simulink model "ACDCMG_woPV"  (R2020b)
settings: Solver=FixedStepAuto  StartTime=0.0  StopTime=0.2  FixedStep=Ts  MaxStep=1e-2  RelTol=1e-3
InitFcn:
  | Set_parameters_R2018
undefined symbols (not defined in the file): D1, D_invs, Delta, dis11, dis14, dis2, dis3, dis4, dis5, dis6, dis8, DiscIntNeverNeededParam, ee_sli_rtmsupport, fn, Fnom, gcbh, H_invs, Ion, Lithium, max_min, P_Load_3, P_nom_inv, Pnom_T1, Pnom_T2, Pnom_T3, Ql_Load_3, R_Load_9, R_Load_DC, Rl, Rls, S, sigbuilder_block, Ts, Ts_Control, Ts_Power, V1_LL_T3, VnInv, Vnom_DC, Vnom_Diesel, Vnom_prim, Vnom_sec, Vnom_ter_AC_DC, Xl, Xls
libraries: powerlib x238, powerlib_meascontrol x103, powerlib_extras x55, simulink x21, pid_lib x4, eeGeneralControl x2, re_lib x1, electricdrivelib x1, eeSinusoidalMeasurementV2 x1, eePowerMeasurement x1
(part 7 of 9)

== system ACDCMG_woPV/Inverter 300 (DC) // 150 V (AC) P_nom 3kW4/Control of Inverter/Positive-Sequence Active & Reactive Power1 ==
  note: Discrete 3-phase Positive-Sequence Active & Reactive Power
  note: Pierre Giroux, Gilbert Sybille
      | Power System Simulation Laboratory
      | IREQ, Hydro-Quebc
  Vabc : Inport  PortDimensions=3
  Iabc : Inport  Port=2  PortDimensions=3
  Deg->Rad : Gain  Gain=pi/180  SaturateOnIntegerOverflow=on  OutDataTypeStr=Inherit: Same as input  ParamDataTypeStr=Inherit: Same as input
  Discrete 3-phase Positive-Sequence Fundamental Value (I) : powerlib_extras/Discrete Measurements/Discrete 3-phase Positive-Sequence Fundamental Value  Freq=Freq  Par_Init=Par_Iinit  Ts=Ts
      settings: SourceProductBaseCode=PS
  Discrete 3-phase Positive-Sequence Fundamental Value (V) : powerlib_extras/Discrete Measurements/Discrete 3-phase Positive-Sequence Fundamental Value  Freq=Freq  Par_Init=Par_Vinit  Ts=Ts
      settings: SourceProductBaseCode=PS
  Gain1 : Gain  Gain=3/2  SaturateOnIntegerOverflow=on  OutDataTypeStr=Inherit: Same as input  ParamDataTypeStr=Inherit: Same as input
  Mag->RMS : Gain  Gain=1/sqrt(2)
  Mux1 : Mux  Inputs=2
  Mux2 : Mux  Inputs=2
  Mux3 : Mux  Inputs=2
  Product : Product  InputSameDT=on  SaturateOnIntegerOverflow=on  OutDataTypeStr=Inherit: Same as first input
  Product1 : Product  InputSameDT=on  SaturateOnIntegerOverflow=on  OutDataTypeStr=Inherit: Same as first input
  Product2 : Product  InputSameDT=on  SaturateOnIntegerOverflow=on  OutDataTypeStr=Inherit: Same as first input
  Sum : Sum  Inputs=+-  InputSameDT=on  SaturateOnIntegerOverflow=on  OutDataTypeStr=Inherit: Same as first input
  Trigonometric Function : Trigonometry
  Trigonometric Function1 : Trigonometry  Operator=cos
  W->kW Var->kvar : Gain  Gain=1/1000
  RMS_V_I : Outport
  P_Q(kW) : Outport  Port=2
  Phase_V_I : Outport  Port=3
  PF : Outport  Port=4
  wires:
  Vabc/1 -> Discrete 3-phase Positive-Sequence Fundamental Value (V)/1
  Iabc/1 -> Discrete 3-phase Positive-Sequence Fundamental Value (I)/1
  Discrete 3-phase Positive-Sequence Fundamental Value (V)/2 -> Sum/1, Mux1/1
  Discrete 3-phase Positive-Sequence Fundamental Value (I)/2 -> Sum/2, Mux1/2
  Sum/1 -> Deg->Rad/1
  Deg->Rad/1 -> Trigonometric Function1/1, Trigonometric Function/1
  Trigonometric Function1/1 -> PF/1, Product/2
  Trigonometric Function/1 -> Product1/1
  Mux2/1 -> Gain1/1
  Product/1 -> Mux2/1
  Product1/1 -> Mux2/2
  Product2/1 -> Product/1, Product1/2
  Discrete 3-phase Positive-Sequence Fundamental Value (V)/1 -> Mux3/1, Product2/1
  Discrete 3-phase Positive-Sequence Fundamental Value (I)/1 -> Mux3/2, Product2/2
  Mux1/1 -> Phase_V_I/1
  Mux3/1 -> Mag->RMS/1
  Mag->RMS/1 -> RMS_V_I/1
  Gain1/1 -> W->kW Var->kvar/1
  W->kW Var->kvar/1 -> P_Q(kW)/1

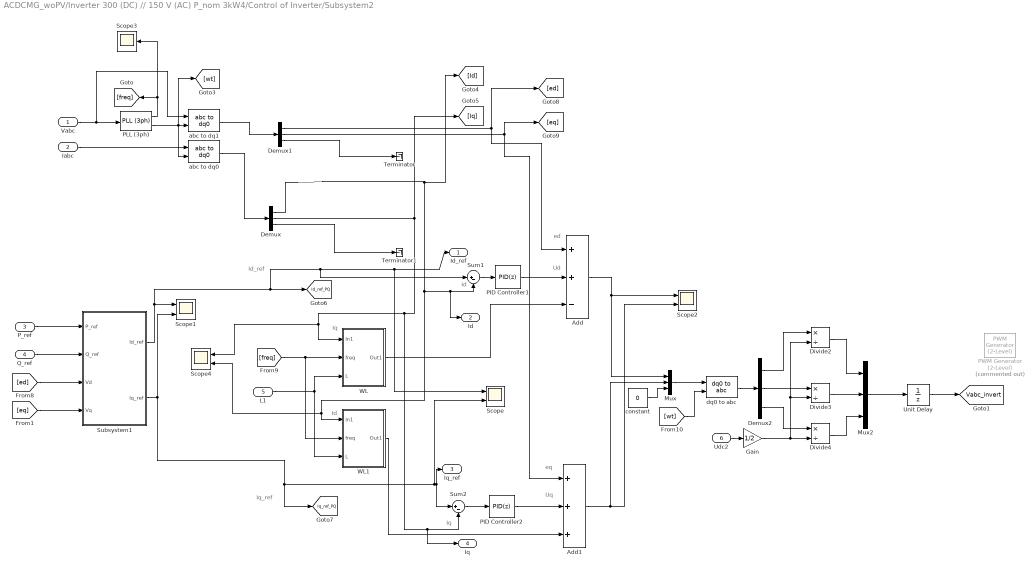
== system ACDCMG_woPV/Inverter 300 (DC) // 150 V (AC) P_nom 3kW4/Control of Inverter/Subsystem2 ==
  note: Iq_ref
  note: Id
  note: Id_ref
  note: Ud
  note: Uq
  note: eq
  note: ed
  note: Iq
  note: Id
  note: Iq
  Vabc : Inport
  Iabc : Inport  Port=2
  P_ref : Inport  Port=3
  Q_ref : Inport  Port=4
  L1 : Inport  Port=5
  Udc2 : Inport  Port=6
  Add : Sum  Inputs=++-
  Add1 : Sum  Inputs=+++
  Demux : Demux  Outputs=3
  Demux1 : Demux  Outputs=3
  Demux2 : Demux  Outputs=3
  Divide2 : Product  Inputs=*/
  Divide3 : Product  Inputs=*/
  Divide4 : Product  Inputs=*/
  Gain : Gain  Gain=1/2
  Mux : Mux  Inputs=3
  Mux2 : Mux  Inputs=3
  PID Controller1 : pid_lib/PID Controller  Controller=PID  Form=Parallel  TimeDomain=Discrete-time  UseExternalTs=off  SampleTime=Ts_Control  IntegratorMethod=Forward Euler  FilterMethod=Forward Euler  ControllerParametersSource=internal  P=Kp  I=Ki  D=Kd  N=100  UseFilter=on  TunerSelectOption=Transfer Function Based (PID Tuner App)  InitialConditionSource=internal  InitialConditionForIntegrator=0  InitialConditionForFilter=0  DifferentiatorICPrevScaledInput=0  ExternalReset=none  TrackingMode=off  Kt=1  LimitOutput=off  SatLimitsSource=internal  UpperSaturationLimit=inf  LowerSaturationLimit=-inf  LinearizeAsGain=on  AntiWindupMode=none  Kb=1  POutMin=[]  POutMax=[]  IOutMin=[]  IOutMax=[]  DOutMin=[]  DOutMax=[]  NOutMin=[]  NOutMax=[]  SumOutMin=[]  SumOutMax=[]  SaturationOutMin=[]  SaturationOutMax=[]  PParamMin=[]  PParamMax=[]  IParamMin=[]  IParamMax=[]  DParamMin=[]  DParamMax=[]  NParamMin=[]  NParamMax=[]  KbParamMin=[]  KbParamMax=[]  KtParamMin=[]  KtParamMax=[]  KbOutMin=[]  KbOutMax=[]  KtOutMin=[]  KtOutMax=[]  IntegratorOutMin=[]  IntegratorOutMax=[]  FilterOutMin=[]  FilterOutMax=[]  SumI1OutMin=[]  SumI1OutMax=[]  SumI2OutMin=[]  SumI2OutMax=[]  SumI3OutMin=[]  SumI3OutMax=[]  SumI4OutMin=[]  SumI4OutMax=[]  SumDOutMin=[]  SumDOutMax=[]  DifferentiatorOutMin=[]  DifferentiatorOutMax=[]  FilterDiffOutCoefMin=[]  FilterDiffOutCoefMax=[]  ReciprocalOutMin=[]  ReciprocalOutMax=[]  SumDenOutMin=[]  SumDenOutMax=[]  SumNumOutMin=[]  SumNumOutMax=[]  DivideOutMin=[]  DivideOutMax=[]  UdiffTsProdOutMin=[]  UdiffTsProdOutMax=[]  NTsProdOutMin=[]  NTsProdOutMax=[]  UintegralTsProdOutMin=[]  UintegralTsProdOutMax=[]  UngainTsProdOutMin=[]  UngainTsProdOutMax=[]  IntegratorContinuousStateAttributes=''  IntegratorStateMustResolveToSignalObject=off  IntegratorRTWStateStorageClass=Auto  FilterContinuousStateAttributes=''  FilterStateMustResolveToSignalObject=off  FilterRTWStateStorageClass=Auto  ParallelPVariant=InternalParameters  IdealPVariant=Disabled  IVariant=InternalParameters  DVariant=InternalParameters  IntegratorVariant=Discrete  SatVariant=Disabled  AWVariant=Passthrough  PCopyVariant=Disabled  TRVariant=Disabled  FdbkBlocksVariant=Forward  IdealPFdbkVariant=Disabled  SatFdbkVariant=Disabled  DerivativeFilterVariant=ForwardEulerFilter  NVariant=InternalParameters  NCopyVariant=Disabled  FilterICVariant=InternalICsFilter  IntegratorICVariant=InternalICs  ExternalResetVariant=Disabled  TRSumVariant=Passthrough  SumFdbkVariant=Disabled  SumVariant=Sum_PID  TsampFilterVariant=InternalTs  TsampNgainVariant=Passthrough  TsampIntegralVariant=Passthrough  ExternalSaturationOutDataTypeStr=Inherit: Same as second input
  PID Controller2 : pid_lib/PID Controller  Controller=PID  Form=Parallel  TimeDomain=Discrete-time  UseExternalTs=off  SampleTime=Ts_Control  IntegratorMethod=Forward Euler  FilterMethod=Forward Euler  ControllerParametersSource=internal  P=Kp  I=Ki  D=Kd  N=100  UseFilter=on  TunerSelectOption=Transfer Function Based (PID Tuner App)  InitialConditionSource=internal  InitialConditionForIntegrator=0  InitialConditionForFilter=0  DifferentiatorICPrevScaledInput=0  ExternalReset=none  TrackingMode=off  Kt=1  LimitOutput=off  SatLimitsSource=internal  UpperSaturationLimit=inf  LowerSaturationLimit=-inf  LinearizeAsGain=on  AntiWindupMode=none  Kb=1  POutMin=[]  POutMax=[]  IOutMin=[]  IOutMax=[]  DOutMin=[]  DOutMax=[]  NOutMin=[]  NOutMax=[]  SumOutMin=[]  SumOutMax=[]  SaturationOutMin=[]  SaturationOutMax=[]  PParamMin=[]  PParamMax=[]  IParamMin=[]  IParamMax=[]  DParamMin=[]  DParamMax=[]  NParamMin=[]  NParamMax=[]  KbParamMin=[]  KbParamMax=[]  KtParamMin=[]  KtParamMax=[]  KbOutMin=[]  KbOutMax=[]  KtOutMin=[]  KtOutMax=[]  IntegratorOutMin=[]  IntegratorOutMax=[]  FilterOutMin=[]  FilterOutMax=[]  SumI1OutMin=[]  SumI1OutMax=[]  SumI2OutMin=[]  SumI2OutMax=[]  SumI3OutMin=[]  SumI3OutMax=[]  SumI4OutMin=[]  SumI4OutMax=[]  SumDOutMin=[]  SumDOutMax=[]  DifferentiatorOutMin=[]  DifferentiatorOutMax=[]  FilterDiffOutCoefMin=[]  FilterDiffOutCoefMax=[]  ReciprocalOutMin=[]  ReciprocalOutMax=[]  SumDenOutMin=[]  SumDenOutMax=[]  SumNumOutMin=[]  SumNumOutMax=[]  DivideOutMin=[]  DivideOutMax=[]  UdiffTsProdOutMin=[]  UdiffTsProdOutMax=[]  NTsProdOutMin=[]  NTsProdOutMax=[]  UintegralTsProdOutMin=[]  UintegralTsProdOutMax=[]  UngainTsProdOutMin=[]  UngainTsProdOutMax=[]  IntegratorContinuousStateAttributes=''  IntegratorStateMustResolveToSignalObject=off  IntegratorRTWStateStorageClass=Auto  FilterContinuousStateAttributes=''  FilterStateMustResolveToSignalObject=off  FilterRTWStateStorageClass=Auto  ParallelPVariant=InternalParameters  IdealPVariant=Disabled  IVariant=InternalParameters  DVariant=InternalParameters  IntegratorVariant=Discrete  SatVariant=Disabled  AWVariant=Passthrough  PCopyVariant=Disabled  TRVariant=Disabled  FdbkBlocksVariant=Forward  IdealPFdbkVariant=Disabled  SatFdbkVariant=Disabled  DerivativeFilterVariant=ForwardEulerFilter  NVariant=InternalParameters  NCopyVariant=Disabled  FilterICVariant=InternalICsFilter  IntegratorICVariant=InternalICs  ExternalResetVariant=Disabled  TRSumVariant=Passthrough  SumFdbkVariant=Disabled  SumVariant=Sum_PID  TsampFilterVariant=InternalTs  TsampNgainVariant=Passthrough  TsampIntegralVariant=Passthrough  ExternalSaturationOutDataTypeStr=Inherit: Same as second input
  PLL (3ph) : powerlib_meascontrol/PLL/PLL (3ph)  Fmin=59.5  Par_Init=[0, 60]  ParK=[180, 3200, 1]  TcD=1e-4  MaxRateChangeFreq=12  FilterCutOffFreq=25  Ts=Ts_Control  AGC=on
  PWM Generator (2-Level) : powerlib_meascontrol/Pulse & Signal Generators/PWM Generator (2-Level)  Commented=on  ModulatorType=Three-phase bridge (6 pulses)  ModulatorMode=Unsynchronized  Fc=15000  Pc=90  nF=27  MinMax="[ -1  1 ]"  SamplingTechnique=Natural  ModulatingSignals=off  m=0.8  Freq=60  Phase=0  Ts=Ts_Power  ShowCarrierOutport=off
  Scope{,1..2,4} (4 alike) : Scope  NumInputPorts=2
  Scope3 : Scope
  Subsystem1 : Subsystem
  Sum1 : Sum  Inputs=|+-
  Sum2 : Sum  Inputs=|+-
  Terminator : Terminator
  Terminator1 : Terminator
  Unit Delay : UnitDelay  SampleTime=-1  HasFrameUpgradeWarning=on
  WL : Subsystem
  WL1 : Subsystem
  abc to dq0 : powerlib_meascontrol/Transformations/abc to dq0  Alignment=90 degrees behind phase A axis
  abc to dq1 : powerlib_meascontrol/Transformations/abc to dq0  Alignment=90 degrees behind phase A axis
  constant : Constant  Value=0
  dq0 to abc : powerlib_meascontrol/Transformations/dq0 to abc  Alignment=90 degrees behind phase A axis
  Id_ref : Outport
  Id : Outport  Port=2
  Iq_ref : Outport  Port=3
  Iq : Outport  Port=4
  tag scope: Id_ref_PQ=global, Iq_ref_PQ=global, Vabc_invert=global
  wires:
  abc to dq1/1 -> Demux1/1
  Sum1/1 -> PID Controller1/1
  Iabc/1 -> abc to dq0/1
  Vabc/1 -> abc to dq1/1, PLL (3ph)/1
  PLL (3ph)/2 -> [wt], abc to dq1/2, abc to dq0/2
  Demux1/1 -> Add/1, [ed]
  L1/1 -> WL/3(L), WL1/3(L)
  WL/1(Out1) -> Add/3
  [freq] -> WL1/2(freq), WL/2(freq)
  PLL (3ph)/1 -> Scope3/1, [freq]
  Demux2/1 -> Divide2/1
  Add/1 -> Mux/1, Scope2/1
  PID Controller2/1 -> Add1/2
  Sum2/1 -> PID Controller2/1
  Demux2/2 -> Divide3/1
  WL1/1(Out1) -> Add1/3
  Demux1/2 -> Add1/1, [eq]
  Add1/1 -> Mux/2, Scope2/2
  Gain/1 -> Divide3/2, Divide2/2, Divide4/2
  Divide4/1 -> Mux2/3
  Divide2/1 -> Mux2/1
  Mux/1 -> dq0 to abc/1
  Demux2/3 -> Divide4/1
  Divide3/1 -> Mux2/2
  dq0 to abc/1 -> Demux2/1
  PID Controller1/1 -> Add/2
  [wt] -> dq0 to abc/2
  Udc2/1 -> Gain/1
  Demux1/3 -> Terminator/1
  Demux/3 -> Terminator1/1
  constant/1 -> Mux/3
  P_ref/1 -> Subsystem1/1(P_ref)
  Q_ref/1 -> Subsystem1/2(Q_ref)
  [ed] -> Subsystem1/3(Vd)
  [eq] -> Subsystem1/4(Vq)
  Subsystem1/2(Iq_ref) -> Scope1/2, [Iq_ref_PQ], Scope/2, Iq_ref/1, Sum2/1
  Subsystem1/1(Id_ref) -> Sum1/1, Scope/1, Id_ref/1, [Id_ref_PQ], Scope1/1
  Demux/1 -> Scope4/2, WL1/1(In1), Id/1, Sum1/2, [Id]
  Demux/2 -> [Iq], Scope4/1, WL/1(In1), Iq/1, Sum2/2
  abc to dq0/1 -> Demux/1
  Mux2/1 -> Unit Delay/1
  Unit Delay/1 -> [Vabc_invert]

== system ACDCMG_woPV/Inverter 300 (DC) // 150 V (AC) P_nom 3kW4/Control of Inverter/V//F ==
  e : Inport
  io : Inport  Port=2
  i : Inport  Port=3
  Udc : Inport  Port=4
  Constant : Constant  Value=150*sqrt(2)
  Constant1 : Constant  Value=0
  Constant2 : Constant  Commented=on
  Constant3 : Constant  Commented=on
  Constant4 : Constant
  From : From  Commented=on  GotoTag=P_mea_inv  TagVisibility=global
  Gain : Gain  Commented=on  Gain=1/P_nom_inv
  Gain1 : Gain  Gain=Fnom
  Gain2 : Gain  Commented=on  Gain=-1
  Scope : Scope  NumInputPorts=2
  Subsystem : Subsystem
  Sum : Sum  Commented=on  Inputs=|+-
  Sum1 : Sum  Commented=on  Inputs=|++
  Transfer Fcn : TransferFcn  Commented=on  Denominator=[2*H_invs D_invs]
  UIcontrol : Subsystem
  wires:
  Constant/1 -> UIcontrol/1(ed_ref)
  Constant1/1 -> UIcontrol/3(eq_ref)
  Udc/1 -> UIcontrol/9(Udc)
  e/1 -> Subsystem/1(e)
  i/1 -> Subsystem/3(i)
  Subsystem/1(ed) -> UIcontrol/2(ed)
  Subsystem/2(eq) -> UIcontrol/4(eq)
  Subsystem/3(iod) -> UIcontrol/5(iod)
  Subsystem/4(ioq) -> UIcontrol/6(ioq)
  Subsystem/8("wt ") -> UIcontrol/8("wt ")
  Subsystem/7(w) -> UIcontrol/7(w)
  Subsystem/5(id) -> UIcontrol/11(id)
  Subsystem/6(iq) -> UIcontrol/10(iq)
  io/1 -> Subsystem/2(io)
  From/1 -> Gain/1
  Gain1/1 -> Scope/1, Subsystem/4(fcmd)
  Gain/1 -> Scope/2, Sum/1
  Constant2/1 -> Sum/2
  Sum/1 -> Gain2/1
  Gain2/1 -> Transfer Fcn/1
  Transfer Fcn/1 -> Sum1/1
  Constant3/1 -> Sum1/2
  Constant4/1 -> Gain1/1

== system ACDCMG_woPV/Grid Bi-directional Converter 1.1 300 (DC) // 150 V (AC) P_nom 3kW/Control of Inverter/MI Controller/OP max // min ==
  note: DC to AC
  note: AC to DC
  Constant2 : Constant  Value=max_min
  OP_max1 : Constant  Value=1.2
  OP_min1 : Constant
  Switch2 : Switch  Criteria=u2 > Threshold
  ctrl : Outport  VectorParamsAs1DForOutWhenUnconnected=off
  wires:
  OP_max1/1 -> Switch2/1
  OP_min1/1 -> Switch2/3
  Constant2/1 -> Switch2/2
  Switch2/1 -> ctrl/1

== system ACDCMG_woPV/Grid Bi-directional Converter 1.1 300 (DC) // 150 V (AC) P_nom 3kW/Control of Inverter/MI Controller/Subsystem ==
  sin_cos : Inport  PortDimensions=2
  Demux : Demux  Outputs=2
      settings: DisplayOption=none
  Fcn2 : Fcn  Expr=1*u[1]
  Fcn4 : Fcn  Expr=1*u[3]
  Fcn5 : Fcn  Expr=1*u[5]
  K1 : Constant  Value=0.5
  K2 : Constant  Value=sqrt(3)/2
  Mux2 : Mux  Inputs=6
  Product{,1..3} (4 alike) : Product  InputSameDT=on  SaturateOnIntegerOverflow=on  OutDataTypeStr=Inherit: Same as first input
  Sum : Sum  Inputs=--  InputSameDT=on  SaturateOnIntegerOverflow=on  OutDataTypeStr=Inherit: Same as first input
  Sum1 : Sum  Inputs=-+  InputSameDT=on  SaturateOnIntegerOverflow=on  OutDataTypeStr=Inherit: Same as first input
  Sum2 : Sum  Inputs=--  InputSameDT=on  SaturateOnIntegerOverflow=on  OutDataTypeStr=Inherit: Same as first input
  Sum3 : Sum  Inputs=--  InputSameDT=on  SaturateOnIntegerOverflow=on  OutDataTypeStr=Inherit: Same as first input
  Va : Outport  VectorParamsAs1DForOutWhenUnconnected=off
  Vb : Outport  Port=2  VectorParamsAs1DForOutWhenUnconnected=off
  Vc : Outport  Port=3  VectorParamsAs1DForOutWhenUnconnected=off
  wires:
  sin_cos/1 -> Demux/1
  Demux/1 -> Product/1, Product2/1, Sum2/2, Mux2/1  "sin(wt)"
  Product/1 -> Sum/1
  Product1/1 -> Sum/2
  Product3/1 -> Sum1/1
  Product2/1 -> Sum1/2
  Sum3/1 -> Mux2/6  "cos(wt+2pi/3)"
  Sum2/1 -> Mux2/5  "sin(wt+2pi/3)"
  K1/1 -> Product/2, Product3/2
  K2/1 -> Product1/2, Product2/2
  Sum/1 -> Mux2/3, Sum2/1  "sin(wt-2pi/3)"
  Sum1/1 -> Mux2/4, Sum3/1  "cos(wt-2pi/3)"
  Demux/2 -> Sum3/2, Product3/1, Product1/1, Mux2/2  "cos(wt)"
  Mux2/1 -> Fcn2/1, Fcn4/1, Fcn5/1
  Fcn2/1 -> Va/1
  Fcn4/1 -> Vb/1
  Fcn5/1 -> Vc/1

== system ACDCMG_woPV/Grid Bi-directional Converter 1.1 300 (DC) // 150 V (AC) P_nom 3kW/Control of Inverter/MI Controller/Subsystem1 ==
  note: AC to DC
  note: DC to AC
  Constant1 : Constant  Value=max_min
  Constant2 : Constant  Value=2*pi
  Deg->Rad : Gain  Gain=pi/180  SaturateOnIntegerOverflow=on  OutDataTypeStr=Inherit: Same as input  ParamDataTypeStr=Inherit: Same as input
  Freq1 : Constant  Value=Fnom
  Freq2 : Constant  Value=2*pi
  Math Function : Math  Operator=mod  SignedPower=on  SaturateOnIntegerOverflow=on
  Mux5 : Mux  Inputs=2
  OP_max1 : Constant  Value=0
  OP_min1 : Constant  Value=228
  Product7 : Product  Inputs=***  InputSameDT=on  SaturateOnIntegerOverflow=on  OutDataTypeStr=Inherit: Same as first input
  Sum : Sum  InputSameDT=on  SaturateOnIntegerOverflow=on  OutDataTypeStr=Inherit: Same as first input
  Switch2 : Switch  Criteria=u2 > Threshold
  Trigonometric Function : Trigonometry
  Trigonometric Function1 : Trigonometry  Operator=cos
  t : DigitalClock  SampleTime=Ts
  Frec : Outport  VectorParamsAs1DForOutWhenUnconnected=off
  sin_cos : Outport  Port=2  VectorParamsAs1DForOutWhenUnconnected=off
  wt : Outport  Port=3  VectorParamsAs1DForOutWhenUnconnected=off
  wires:
  Switch2/1 -> Deg->Rad/1
  Deg->Rad/1 -> Sum/2
  Freq1/1 -> Frec/1, Product7/1
  Trigonometric Function/1 -> Mux5/1
  Sum/1 -> Math Function/1
  Trigonometric Function1/1 -> Mux5/2
  Product7/1 -> Sum/1
  Freq2/1 -> Product7/3
  Constant2/1 -> Math Function/2
  t/1 -> Product7/2
  Math Function/1 -> wt/1, Trigonometric Function1/1, Trigonometric Function/1
  Mux5/1 -> sin_cos/1
  Constant1/1 -> Switch2/2
  OP_max1/1 -> Switch2/1
  OP_min1/1 -> Switch2/3

== system ACDCMG_woPV/Grid Bi-directional Converter 1.1 300 (DC) // 150 V (AC) P_nom 3kW1/Control of Inverter/MI Controller/OP max // min ==
  note: DC to AC
  note: AC to DC
  Constant2 : Constant  Value=max_min
  OP_max1 : Constant  Value=1.2
  OP_min1 : Constant
  Switch2 : Switch  Criteria=u2 > Threshold
  ctrl : Outport  VectorParamsAs1DForOutWhenUnconnected=off
  wires:
  OP_max1/1 -> Switch2/1
  OP_min1/1 -> Switch2/3
  Constant2/1 -> Switch2/2
  Switch2/1 -> ctrl/1

== system ACDCMG_woPV/Grid Bi-directional Converter 1.1 300 (DC) // 150 V (AC) P_nom 3kW1/Control of Inverter/MI Controller/Subsystem ==
  sin_cos : Inport  PortDimensions=2
  Demux : Demux  Outputs=2
      settings: DisplayOption=none
  Fcn2 : Fcn  Expr=1*u[1]
  Fcn4 : Fcn  Expr=1*u[3]
  Fcn5 : Fcn  Expr=1*u[5]
  K1 : Constant  Value=0.5
  K2 : Constant  Value=sqrt(3)/2
  Mux2 : Mux  Inputs=6
  Product{,1..3} (4 alike) : Product  InputSameDT=on  SaturateOnIntegerOverflow=on  OutDataTypeStr=Inherit: Same as first input
  Sum : Sum  Inputs=--  InputSameDT=on  SaturateOnIntegerOverflow=on  OutDataTypeStr=Inherit: Same as first input
  Sum1 : Sum  Inputs=-+  InputSameDT=on  SaturateOnIntegerOverflow=on  OutDataTypeStr=Inherit: Same as first input
  Sum2 : Sum  Inputs=--  InputSameDT=on  SaturateOnIntegerOverflow=on  OutDataTypeStr=Inherit: Same as first input
  Sum3 : Sum  Inputs=--  InputSameDT=on  SaturateOnIntegerOverflow=on  OutDataTypeStr=Inherit: Same as first input
  Va : Outport  VectorParamsAs1DForOutWhenUnconnected=off
  Vb : Outport  Port=2  VectorParamsAs1DForOutWhenUnconnected=off
  Vc : Outport  Port=3  VectorParamsAs1DForOutWhenUnconnected=off
  wires:
  sin_cos/1 -> Demux/1
  Demux/1 -> Product/1, Product2/1, Sum2/2, Mux2/1  "sin(wt)"
  Product/1 -> Sum/1
  Product1/1 -> Sum/2
  Product3/1 -> Sum1/1
  Product2/1 -> Sum1/2
  Sum3/1 -> Mux2/6  "cos(wt+2pi/3)"
  Sum2/1 -> Mux2/5  "sin(wt+2pi/3)"
  K1/1 -> Product/2, Product3/2
  K2/1 -> Product1/2, Product2/2
  Sum/1 -> Mux2/3, Sum2/1  "sin(wt-2pi/3)"
  Sum1/1 -> Mux2/4, Sum3/1  "cos(wt-2pi/3)"
  Demux/2 -> Sum3/2, Product3/1, Product1/1, Mux2/2  "cos(wt)"
  Mux2/1 -> Fcn2/1, Fcn4/1, Fcn5/1
  Fcn2/1 -> Va/1
  Fcn4/1 -> Vb/1
  Fcn5/1 -> Vc/1

== system ACDCMG_woPV/Grid Bi-directional Converter 1.1 300 (DC) // 150 V (AC) P_nom 3kW1/Control of Inverter/MI Controller/Subsystem1 ==
  note: AC to DC
  note: DC to AC
  Constant1 : Constant  Value=max_min
  Constant2 : Constant  Value=2*pi
  Deg->Rad : Gain  Gain=pi/180  SaturateOnIntegerOverflow=on  OutDataTypeStr=Inherit: Same as input  ParamDataTypeStr=Inherit: Same as input
  Freq1 : Constant  Value=Fnom
  Freq2 : Constant  Value=2*pi
  Math Function : Math  Operator=mod  SignedPower=on  SaturateOnIntegerOverflow=on
  Mux5 : Mux  Inputs=2
  OP_max1 : Constant  Value=0
  OP_min1 : Constant  Value=228
  Product7 : Product  Inputs=***  InputSameDT=on  SaturateOnIntegerOverflow=on  OutDataTypeStr=Inherit: Same as first input
  Sum : Sum  InputSameDT=on  SaturateOnIntegerOverflow=on  OutDataTypeStr=Inherit: Same as first input
  Switch2 : Switch  Criteria=u2 > Threshold
  Trigonometric Function : Trigonometry
  Trigonometric Function1 : Trigonometry  Operator=cos
  t : DigitalClock  SampleTime=Ts
  Frec : Outport  VectorParamsAs1DForOutWhenUnconnected=off
  sin_cos : Outport  Port=2  VectorParamsAs1DForOutWhenUnconnected=off
  wt : Outport  Port=3  VectorParamsAs1DForOutWhenUnconnected=off
  wires:
  Switch2/1 -> Deg->Rad/1
  Deg->Rad/1 -> Sum/2
  Freq1/1 -> Frec/1, Product7/1
  Trigonometric Function/1 -> Mux5/1
  Sum/1 -> Math Function/1
  Trigonometric Function1/1 -> Mux5/2
  Product7/1 -> Sum/1
  Freq2/1 -> Product7/3
  Constant2/1 -> Math Function/2
  t/1 -> Product7/2
  Math Function/1 -> wt/1, Trigonometric Function1/1, Trigonometric Function/1
  Mux5/1 -> sin_cos/1
  Constant1/1 -> Switch2/2
  OP_max1/1 -> Switch2/1
  OP_min1/1 -> Switch2/3

== system ACDCMG_woPV/Grid Bi-directional Converter 1.1 300 (DC) // 150 V (AC) P_nom 3kW2/Control of Inverter/MI Controller/OP max // min ==
  note: DC to AC
  note: AC to DC
  Constant2 : Constant  Value=max_min
  OP_max1 : Constant  Value=1.2
  OP_min1 : Constant
  Switch2 : Switch  Criteria=u2 > Threshold
  ctrl : Outport  VectorParamsAs1DForOutWhenUnconnected=off
  wires:
  OP_max1/1 -> Switch2/1
  OP_min1/1 -> Switch2/3
  Constant2/1 -> Switch2/2
  Switch2/1 -> ctrl/1

== system ACDCMG_woPV/Grid Bi-directional Converter 1.1 300 (DC) // 150 V (AC) P_nom 3kW2/Control of Inverter/MI Controller/Subsystem ==
  sin_cos : Inport  PortDimensions=2
  Demux : Demux  Outputs=2
      settings: DisplayOption=none
  Fcn2 : Fcn  Expr=1*u[1]
  Fcn4 : Fcn  Expr=1*u[3]
  Fcn5 : Fcn  Expr=1*u[5]
  K1 : Constant  Value=0.5
  K2 : Constant  Value=sqrt(3)/2
  Mux2 : Mux  Inputs=6
  Product{,1..3} (4 alike) : Product  InputSameDT=on  SaturateOnIntegerOverflow=on  OutDataTypeStr=Inherit: Same as first input
  Sum : Sum  Inputs=--  InputSameDT=on  SaturateOnIntegerOverflow=on  OutDataTypeStr=Inherit: Same as first input
  Sum1 : Sum  Inputs=-+  InputSameDT=on  SaturateOnIntegerOverflow=on  OutDataTypeStr=Inherit: Same as first input
  Sum2 : Sum  Inputs=--  InputSameDT=on  SaturateOnIntegerOverflow=on  OutDataTypeStr=Inherit: Same as first input
  Sum3 : Sum  Inputs=--  InputSameDT=on  SaturateOnIntegerOverflow=on  OutDataTypeStr=Inherit: Same as first input
  Va : Outport  VectorParamsAs1DForOutWhenUnconnected=off
  Vb : Outport  Port=2  VectorParamsAs1DForOutWhenUnconnected=off
  Vc : Outport  Port=3  VectorParamsAs1DForOutWhenUnconnected=off
  wires:
  sin_cos/1 -> Demux/1
  Demux/1 -> Product/1, Product2/1, Sum2/2, Mux2/1  "sin(wt)"
  Product/1 -> Sum/1
  Product1/1 -> Sum/2
  Product3/1 -> Sum1/1
  Product2/1 -> Sum1/2
  Sum3/1 -> Mux2/6  "cos(wt+2pi/3)"
  Sum2/1 -> Mux2/5  "sin(wt+2pi/3)"
  K1/1 -> Product/2, Product3/2
  K2/1 -> Product1/2, Product2/2
  Sum/1 -> Mux2/3, Sum2/1  "sin(wt-2pi/3)"
  Sum1/1 -> Mux2/4, Sum3/1  "cos(wt-2pi/3)"
  Demux/2 -> Sum3/2, Product3/1, Product1/1, Mux2/2  "cos(wt)"
  Mux2/1 -> Fcn2/1, Fcn4/1, Fcn5/1
  Fcn2/1 -> Va/1
  Fcn4/1 -> Vb/1
  Fcn5/1 -> Vc/1

== system ACDCMG_woPV/Grid Bi-directional Converter 1.1 300 (DC) // 150 V (AC) P_nom 3kW2/Control of Inverter/MI Controller/Subsystem1 ==
  note: AC to DC
  note: DC to AC
  Constant1 : Constant  Value=max_min
  Constant2 : Constant  Value=2*pi
  Deg->Rad : Gain  Gain=pi/180  SaturateOnIntegerOverflow=on  OutDataTypeStr=Inherit: Same as input  ParamDataTypeStr=Inherit: Same as input
  Freq1 : Constant  Value=Fnom
  Freq2 : Constant  Value=2*pi
  Math Function : Math  Operator=mod  SignedPower=on  SaturateOnIntegerOverflow=on
  Mux5 : Mux  Inputs=2
  OP_max1 : Constant  Value=0
  OP_min1 : Constant  Value=228
  Product7 : Product  Inputs=***  InputSameDT=on  SaturateOnIntegerOverflow=on  OutDataTypeStr=Inherit: Same as first input
  Sum : Sum  InputSameDT=on  SaturateOnIntegerOverflow=on  OutDataTypeStr=Inherit: Same as first input
  Switch2 : Switch  Criteria=u2 > Threshold
  Trigonometric Function : Trigonometry
  Trigonometric Function1 : Trigonometry  Operator=cos
  t : DigitalClock  SampleTime=Ts
  Frec : Outport  VectorParamsAs1DForOutWhenUnconnected=off
  sin_cos : Outport  Port=2  VectorParamsAs1DForOutWhenUnconnected=off
  wt : Outport  Port=3  VectorParamsAs1DForOutWhenUnconnected=off
  wires:
  Switch2/1 -> Deg->Rad/1
  Deg->Rad/1 -> Sum/2
  Freq1/1 -> Frec/1, Product7/1
  Trigonometric Function/1 -> Mux5/1
  Sum/1 -> Math Function/1
  Trigonometric Function1/1 -> Mux5/2
  Product7/1 -> Sum/1
  Freq2/1 -> Product7/3
  Constant2/1 -> Math Function/2
  t/1 -> Product7/2
  Math Function/1 -> wt/1, Trigonometric Function1/1, Trigonometric Function/1
  Mux5/1 -> sin_cos/1
  Constant1/1 -> Switch2/2
  OP_max1/1 -> Switch2/1
  OP_min1/1 -> Switch2/3

== system ACDCMG_woPV/Grid Bi-directional Converter 1.2 300 (DC) // 150 V (AC) P_nom 3kW/Control of Inverter/MI Controller/Subsystem ==
  sin_cos : Inport  PortDimensions=2
  Demux : Demux  Outputs=2
      settings: DisplayOption=none
  Fcn2 : Fcn  Expr=1*u[1]
  Fcn4 : Fcn  Expr=1*u[3]
  Fcn5 : Fcn  Expr=1*u[5]
  K1 : Constant  Value=0.5
  K2 : Constant  Value=sqrt(3)/2
  Mux2 : Mux  Inputs=6
  Product{,1..3} (4 alike) : Product  InputSameDT=on  SaturateOnIntegerOverflow=on  OutDataTypeStr=Inherit: Same as first input
  Sum : Sum  Inputs=--  InputSameDT=on  SaturateOnIntegerOverflow=on  OutDataTypeStr=Inherit: Same as first input
  Sum1 : Sum  Inputs=-+  InputSameDT=on  SaturateOnIntegerOverflow=on  OutDataTypeStr=Inherit: Same as first input
  Sum2 : Sum  Inputs=--  InputSameDT=on  SaturateOnIntegerOverflow=on  OutDataTypeStr=Inherit: Same as first input
  Sum3 : Sum  Inputs=--  InputSameDT=on  SaturateOnIntegerOverflow=on  OutDataTypeStr=Inherit: Same as first input
  Va : Outport  VectorParamsAs1DForOutWhenUnconnected=off
  Vb : Outport  Port=2  VectorParamsAs1DForOutWhenUnconnected=off
  Vc : Outport  Port=3  VectorParamsAs1DForOutWhenUnconnected=off
  wires:
  sin_cos/1 -> Demux/1
  Demux/1 -> Product/1, Product2/1, Sum2/2, Mux2/1  "sin(wt)"
  Product/1 -> Sum/1
  Product1/1 -> Sum/2
  Product3/1 -> Sum1/1
  Product2/1 -> Sum1/2
  Sum3/1 -> Mux2/6  "cos(wt+2pi/3)"
  Sum2/1 -> Mux2/5  "sin(wt+2pi/3)"
  K1/1 -> Product/2, Product3/2
  K2/1 -> Product1/2, Product2/2
  Sum/1 -> Mux2/3, Sum2/1  "sin(wt-2pi/3)"
  Sum1/1 -> Mux2/4, Sum3/1  "cos(wt-2pi/3)"
  Demux/2 -> Sum3/2, Product3/1, Product1/1, Mux2/2  "cos(wt)"
  Mux2/1 -> Fcn2/1, Fcn4/1, Fcn5/1
  Fcn2/1 -> Va/1
  Fcn4/1 -> Vb/1
  Fcn5/1 -> Vc/1

== system ACDCMG_woPV/Grid Bi-directional Converter 1.2 300 (DC) // 150 V (AC) P_nom 3kW/Control of Inverter/MI Controller/Subsystem1 ==
  CD to AC : Constant  Value=0
  Constant2 : Constant  Value=2*pi
  Deg->Rad : Gain  Gain=pi/180  SaturateOnIntegerOverflow=on  OutDataTypeStr=Inherit: Same as input  ParamDataTypeStr=Inherit: Same as input
  Freq1 : Constant  Value=Fnom
  Freq2 : Constant  Value=2*pi
  Math Function : Math  Operator=mod  SignedPower=on  SaturateOnIntegerOverflow=on
  Mux5 : Mux  Inputs=2
  Product7 : Product  Inputs=***  InputSameDT=on  SaturateOnIntegerOverflow=on  OutDataTypeStr=Inherit: Same as first input
  Sum : Sum  InputSameDT=on  SaturateOnIntegerOverflow=on  OutDataTypeStr=Inherit: Same as first input
  Trigonometric Function : Trigonometry
  Trigonometric Function1 : Trigonometry  Operator=cos
  t : DigitalClock  SampleTime=Ts
  Frec : Outport  VectorParamsAs1DForOutWhenUnconnected=off
  sin_cos : Outport  Port=2  VectorParamsAs1DForOutWhenUnconnected=off
  wt : Outport  Port=3  VectorParamsAs1DForOutWhenUnconnected=off
  wires:
  CD to AC/1 -> Deg->Rad/1
  Deg->Rad/1 -> Sum/2
  Freq1/1 -> Frec/1, Product7/1
  Trigonometric Function/1 -> Mux5/1
  Sum/1 -> Math Function/1
  Trigonometric Function1/1 -> Mux5/2
  Product7/1 -> Sum/1
  Freq2/1 -> Product7/3
  Constant2/1 -> Math Function/2
  t/1 -> Product7/2
  Math Function/1 -> wt/1, Trigonometric Function1/1, Trigonometric Function/1
  Mux5/1 -> sin_cos/1

== system ACDCMG_woPV/Grid Bi-directional Converter 1.2 300 (DC) // 150 V (AC) P_nom 3kW/Control of Inverter/V//F/Subsystem ==
  note: w
  e : Inport
  io : Inport  Port=2
  i : Inport  Port=3
  Constant1 : Constant  Value=2*pi
  Demux : Demux  Outputs=3
  Demux1 : Demux  Outputs=3
  Demux2 : Demux  Outputs=3
  Discrete Virtual PLL : powerlib_extras/Discrete  Control Blocks/Discrete Virtual PLL  Freq=50  Phase=0  Ts=Ts_Control
      settings: SourceProductBaseCode=PS
  Gain1 : Gain  Gain=2*pi
  Integrator : Integrator
  Math Function : Math  Operator=mod  SignedPower=on  SaturateOnIntegerOverflow=on
  Scope : Scope
  Scope3 : Scope
  Terminator{1..4} (4 alike) : Terminator
  abc to dq0 : powerlib_meascontrol/Transformations/abc to dq0  Alignment=90 degrees behind phase A axis
  abc to dq1 : powerlib_meascontrol/Transformations/abc to dq0  Alignment=90 degrees behind phase A axis
  abc to dq2 : powerlib_meascontrol/Transformations/abc to dq0  Alignment=90 degrees behind phase A axis
  abc_to_dq0 Transformation2 : powerlib_extras/Measurements/abc_to_dq0 Transformation
      settings: SourceProductBaseCode=PS
  constant1 : Constant  Value=60
  pack6 Scope1 : Scope  NumInputPorts=2
  ed : Outport
  eq : Outport  Port=2
  iod : Outport  Port=3
  ioq : Outport  Port=4
  id : Outport  Port=5
  iq : Outport  Port=6
  w : Outport  Port=7
  "wt " : Outport  Port=8
  wires:
  e/1 -> abc to dq0/1
  i/1 -> abc to dq1/1
  constant1/1 -> Gain1/1
  Math Function/1 -> Scope3/1, abc to dq1/2, abc to dq2/2, abc to dq0/2, "wt "/1
  abc to dq0/1 -> Demux/1
  Demux1/1 -> id/1
  Demux1/2 -> iq/1
  Demux1/3 -> Terminator3/1
  Demux/1 -> ed/1
  Demux/2 -> eq/1
  Demux/3 -> Terminator1/1
  abc to dq1/1 -> Demux1/1
  Constant1/1 -> Math Function/2
  Integrator/1 -> Math Function/1
  io/1 -> abc to dq2/1
  abc to dq2/1 -> Demux2/1
  Demux2/3 -> Terminator2/1
  Gain1/1 -> Scope/1, w/1, Integrator/1
  Discrete Virtual PLL/2 -> Terminator4/1
  Demux2/1 -> pack6 Scope1/1, iod/1
  Demux2/2 -> pack6 Scope1/2, ioq/1

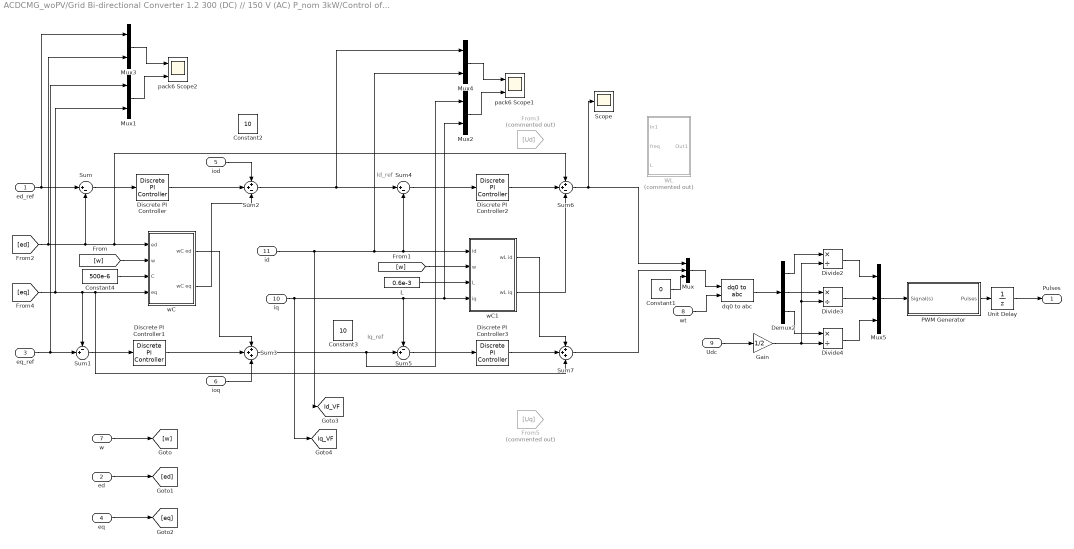
== system ACDCMG_woPV/Grid Bi-directional Converter 1.2 300 (DC) // 150 V (AC) P_nom 3kW/Control of Inverter/V//F/UIcontrol ==
  note: Id_ref
  note: Iq_ref
  ed_ref : Inport
  ed : Inport  Port=2
  eq_ref : Inport  Port=3
  eq : Inport  Port=4
  iod : Inport  Port=5
  ioq : Inport  Port=6
  w : Inport  Port=7
  "wt " : Inport  Port=8
  Udc : Inport  Port=9
  iq : Inport  Port=10
  id : Inport  Port=11
  Constant1 : Constant  Value=0
  Constant2 : Constant  Value=10
  Constant3 : Constant  Value=10
  Constant4 : Constant  Value=500e-6
  Demux2 : Demux  Outputs=3
  Discrete PI Controller : powerlib_extras/Discrete  Control Blocks/Discrete PI Controller  Kp=5  Ki=50  Par_Limits=[1e6 -1e6]  Init=0  Ts=Ts_Control
  Discrete PI Controller1 : powerlib_extras/Discrete  Control Blocks/Discrete PI Controller  Kp=5  Ki=50  Par_Limits=[1e6 -1e6]  Init=0  Ts=Ts_Control
  Discrete PI Controller2 : powerlib_extras/Discrete  Control Blocks/Discrete PI Controller  Kp=25  Ki=1800  Par_Limits=[1e6 -1e6]  Init=0  Ts=Ts_Control
  Discrete PI Controller3 : powerlib_extras/Discrete  Control Blocks/Discrete PI Controller  Kp=25  Ki=1800  Par_Limits=[1e6 -1e6]  Init=0  Ts=Ts_Control
  Divide2 : Product  Inputs=*/
  Divide3 : Product  Inputs=*/
  Divide4 : Product  Inputs=*/
  From3 : From  Commented=on  GotoTag=Ud
  From5 : From  Commented=on  GotoTag=Uq
  Gain : Gain  Gain=1/2
  L : Constant  Value=0.6e-3
  Mux : Mux  Inputs=3
  Mux{1..4} (4 alike) : Mux  Inputs=2
  Mux5 : Mux  Inputs=3
  PWM Generator : Subsystem  AncestorBlock="powerlib_extras/Control  Blocks/PWM Generator"  DialogController=POWERSYS.PowerSysDialog  mask(PWM Generator){GeneratorMode=3-arm  bridge (6 pulses), Fc=10000, Internal=off, mIndex=0.4, Freq=50, Phase=0}
      mask prompts: GeneratorMode "Generator Mode"; Fc "Carrier frequency (Hz):"; Internal "Internal generation of modulating signal(s)"; mIndex "Modulation index  (0<m<1) :"; Freq "Frequency of output voltage (Hz)"; Phase "Phase of output voltage (degrees)"
      mask help:
      | This block generates pulses for carrier-based PWM (Pulse Width Modulation), self-commutated IGBTs,GTOs or FETs bridges.
      |
      | Depending on the number of bridge arms selected in the "Generator Mode" parameter, the block can be used either for single-phase or three-phase PWM control.
      mask init:
      | if Freq==0
      |     Phase=90;
      | end
      | switch GeneratorMode
      | case 1,
      |     Internal_Phase=0;
      |    Signal_PortWidth=1;
      |    Select1_Elements=[1 2];
      |    Select1_PortWidth=2;
      |    Select3_Elements=[1 2];
      |    Select3_PortWidth=4;
      | case 2,
      |     Internal_Phase=0;
      |     Signal_PortWidth=1;
      |     Select1_Elements=[1 2];
      |     Select1_PortWidth=2;
      |     Select3_Elements=[1 2 3 4];
      |     Select3_PortWidth=4;
      | case 3,
      |     Internal_Phase=[0 -2*pi/3 2*pi/3];
      |     Signal_PortWidth=3;
      |     Select1_Elements=[1 4 2 5 3 6];
      |     Select1_PortWidth=6;
      |    Select3_Elements=[1 2 3 4 5 6];
      |    Select3_PortWidth=12;
      | case 4,
      |     Internal_Phase=[0 -2*pi/3 2*pi/3];
      |     Signal_PortWidth=3;
      |     Select1_Elements=[1 4 2 5 3 6];
      |     Select1_PortWidth=6;
      |    Select3_Elements=[1 2 3 4 5 6 7 8 9 10 11 12];
      |    Select3_PortWidth=12;
      | end
      | power_initmask();
      mask Help: web(psbhelp)
      mask TypeOptions GeneratorMode: 1-arm  bridge (2 pulses) | 2-arm  bridge (4 pulses) | 3-arm  bridge (6 pulses) | Double 3-arm  bridges (12 pulses)
      mask Callback Internal: p3=get_param(gcb,'Internal');if strcmp(p3,'on');visible={'on','on','on','on','on','on'};else;visible={'on','on','on','off','off','off'};end;set_param(gcb,'MaskVisibilities',visible)
  Scope : Scope
  Sum : Sum  Inputs=|+-
  Sum1 : Sum  Inputs=-+|
  Sum2 : Sum  Inputs=++-
  Sum3 : Sum  Inputs=+++
  Sum4 : Sum  Inputs=|+-
  Sum5 : Sum  Inputs=-+|
  Sum6 : Sum  Inputs=++-
  Sum7 : Sum  Inputs=+++
  Unit Delay : UnitDelay  SampleTime=-1  HasFrameUpgradeWarning=on
  WL : Subsystem  Commented=on
  dq0 to abc : powerlib_meascontrol/Transformations/dq0 to abc  Alignment=90 degrees behind phase A axis
  pack6 Scope1 : Scope  NumInputPorts=2
  pack6 Scope2 : Scope  NumInputPorts=2
  wC : Subsystem
  wC1 : Subsystem
  Pulses : Outport  VectorParamsAs1DForOutWhenUnconnected=off
  tag scope: Id_VF=global, Iq_VF=global
  wires:
  ed_ref/1 -> Mux3/1, Sum/1
  Sum/1 -> Discrete PI Controller/1
  Mux/1 -> dq0 to abc/1
  "wt "/1 -> dq0 to abc/2
  PWM Generator/1(Pulses) -> Unit Delay/1
  Demux2/1 -> Divide2/1
  Demux2/2 -> Divide3/1
  Gain/1 -> Divide3/2, Divide2/2, Divide4/2
  Divide4/1 -> Mux5/3
  Divide2/1 -> Mux5/1
  Demux2/3 -> Divide4/1
  Divide3/1 -> Mux5/2
  dq0 to abc/1 -> Demux2/1
  Mux5/1 -> PWM Generator/1(Signal(s))
  Udc/1 -> Gain/1
  Constant4/1 -> wC/3(C)
  [w] -> wC/2(w)
  [eq] -> Mux1/2, Sum7/3, wC/4(eq), Sum1/1
  Sum1/1 -> Discrete PI Controller1/1
  eq_ref/1 -> Mux1/1, Sum1/2
  L/1 -> wC1/3(L)
  Sum5/1 -> Discrete PI Controller3/1
  Sum4/1 -> Discrete PI Controller2/1
  Discrete PI Controller3/1 -> Sum7/2
  Discrete PI Controller2/1 -> Sum6/2
  w/1 -> [w]
  [w] -> wC1/2(w)
  ed/1 -> [ed]
  eq/1 -> [eq]
  Sum6/1 -> Scope/1, Mux/1
  Sum7/1 -> Mux/2
  Constant1/1 -> Mux/3
  Mux4/1 -> pack6 Scope1/1
  Mux2/1 -> pack6 Scope1/2
  iq/1 -> [Iq_VF], Sum5/1, wC1/4(iq), Mux2/2
  Discrete PI Controller/1 -> Sum2/2
  Discrete PI Controller1/1 -> Sum3/2
  id/1 -> [Id_VF], Mux4/2, wC1/1(id), Sum4/2
  Mux3/1 -> pack6 Scope2/1
  Mux1/1 -> pack6 Scope2/2
  wC/1(wC ed) -> Sum3/1
  ioq/1 -> Sum3/3
  iod/1 -> Sum2/1
  wC/2(wC eq) -> Sum2/3
  wC1/1(wL id) -> Sum7/1
  wC1/2(wL iq) -> Sum6/3
  [ed] -> Sum6/1, wC/1(ed), Sum/2, Mux3/2
  Sum2/1 -> Mux4/1, Sum4/1
  Sum3/1 -> Mux2/1, Sum5/2
  Unit Delay/1 -> Pulses/1

== system ACDCMG_woPV/Grid Bi-directional Converter 1.2 300 (DC) // 150 V (AC) P_nom 3kW1/Control of Inverter/Subsystem2/Subsystem1 ==
  note: Iq* = 2/3*( P*Vq - Q*Vd ) / ( Vd^2 + Vq^2 )
  note: Reference computation:
  note: Id* = 2/3* ( P*Vd + Q*Vq ) / ( Vd^2 + Vq^2 )
  P_ref : Inport  PortDimensions=1
  Q_ref : Inport  Port=2  PortDimensions=1
  Vd : Inport  Port=3  PortDimensions=1
  Vq : Inport  Port=4  PortDimensions=1
  Constant1 : Constant  Commented=on  Value=0
  Demux3 : Demux  Outputs=2
      settings: DisplayOption=none
  Fcn3 : Fcn  Expr=u(1)*u(1)+u(2)*u(2)
  Gain : Gain  Gain=2/3
  Mux1 : Mux  Inputs=2
  Mux3 : Mux  Inputs=2
  Product{2..5} (4 alike) : Product  InputSameDT=on  SaturateOnIntegerOverflow=on  OutDataTypeStr=Inherit: Same as first input
  Product6 : Product  Inputs=*/  InputSameDT=on  SaturateOnIntegerOverflow=on  OutDataTypeStr=Inherit: Same as first input
  Scope3 : Scope  NumInputPorts=2
  Sum : Sum  InputSameDT=on  SaturateOnIntegerOverflow=on  OutDataTypeStr=Inherit: Same as first input
  Sum1 : Sum  Inputs=+-  InputSameDT=on  SaturateOnIntegerOverflow=on  OutDataTypeStr=Inherit: Same as first input
  Terminator : Terminator  Commented=on
  Id_ref : Outport
  Iq_ref : Outport  Port=2
  wires:
  Vq/1 -> Mux1/2, Product4/2, Product3/1
  Demux3/1 -> Scope3/1, Id_ref/1
  Mux1/1 -> Fcn3/1
  Product3/1 -> Sum/2
  Mux3/1 -> Gain/1
  Vd/1 -> Mux1/1, Product5/2, Product2/1
  Product4/1 -> Sum1/1
  Product6/1 -> Demux3/1
  Fcn3/1 -> Product6/2
  Demux3/2 -> Scope3/2, Iq_ref/1
  P_ref/1 -> Product2/2, Product4/1
  Gain/1 -> Product6/1
  Product2/1 -> Sum/1
  Q_ref/1 -> Product5/1, Product3/2
  Sum1/1 -> Mux3/2
  Product5/1 -> Sum1/2
  Sum/1 -> Mux3/1

== system ACDCMG_woPV/Grid Bi-directional Converter 1.2 300 (DC) // 150 V (AC) P_nom 3kW1/Control of Inverter/Subsystem2/WL ==
  In1 : Inport
  freq : Inport  Port=2
  L : Inport  Port=3
  2pai : Constant  Value=2*pi
  Product : Product  Inputs=**
  Product1 : Product  Inputs=***
  Out1 : Outport
  wires:
  2pai/1 -> Product/2
  L/1 -> Product1/3
  freq/1 -> Product/1
  Product1/1 -> Out1/1
  Product/1 -> Product1/2
  In1/1 -> Product1/1

== system ACDCMG_woPV/Grid Bi-directional Converter 1.2 300 (DC) // 150 V (AC) P_nom 3kW1/Control of Inverter/Subsystem2/WL1 ==
  In1 : Inport
  freq : Inport  Port=2
  L : Inport  Port=3
  2pai : Constant  Value=2*pi
  Product : Product
  Product1 : Product  Inputs=3
  Out1 : Outport
  wires:
  2pai/1 -> Product/2
  L/1 -> Product1/3
  freq/1 -> Product/1
  Product1/1 -> Out1/1
  Product/1 -> Product1/2
  In1/1 -> Product1/1

== system ACDCMG_woPV/Grid Bi-directional Converter 1.2 300 (DC) // 150 V (AC) P_nom 3kW1/Control of Inverter/V//F/Subsystem ==
  note: w
  e : Inport
  io : Inport  Port=2
  i : Inport  Port=3
  fcmd : Inport  Port=4
  Constant1 : Constant  Value=2*pi
  Demux : Demux  Outputs=3
  Demux1 : Demux  Outputs=3
  Demux2 : Demux  Outputs=3
  Discrete Virtual PLL : powerlib_extras/Discrete  Control Blocks/Discrete Virtual PLL  Commented=on  Freq=50  Phase=0  Ts=Ts_Control
      settings: SourceProductBaseCode=PS
  Gain1 : Gain  Gain=2*pi
  Integrator : Integrator
  Math Function : Math  Operator=mod  SignedPower=on  SaturateOnIntegerOverflow=on
  Scope : Scope
  Scope3 : Scope
  Terminator1 : Terminator
  Terminator2 : Terminator
  Terminator3 : Terminator
  Terminator4 : Terminator  Commented=on
  abc to dq0 : powerlib_meascontrol/Transformations/abc to dq0  Alignment=90 degrees behind phase A axis
  abc to dq1 : powerlib_meascontrol/Transformations/abc to dq0  Alignment=90 degrees behind phase A axis
  abc to dq2 : powerlib_meascontrol/Transformations/abc to dq0  Alignment=90 degrees behind phase A axis
  abc_to_dq0 Transformation2 : powerlib_extras/Measurements/abc_to_dq0 Transformation  Commented=on
      settings: SourceProductBaseCode=PS
  pack6 Scope1 : Scope  NumInputPorts=2
  ed : Outport
  eq : Outport  Port=2
  iod : Outport  Port=3
  ioq : Outport  Port=4
  id : Outport  Port=5
  iq : Outport  Port=6
  w : Outport  Port=7
  "wt " : Outport  Port=8
  wires:
  e/1 -> abc to dq0/1
  i/1 -> abc to dq1/1
  fcmd/1 -> Gain1/1
  Math Function/1 -> Scope3/1, abc to dq1/2, abc to dq2/2, abc to dq0/2, "wt "/1
  abc to dq0/1 -> Demux/1
  Demux1/1 -> id/1
  Demux1/2 -> iq/1
  Demux1/3 -> Terminator3/1
  Demux/1 -> ed/1
  Demux/2 -> eq/1
  Demux/3 -> Terminator1/1
  abc to dq1/1 -> Demux1/1
  Constant1/1 -> Math Function/2
  Integrator/1 -> Math Function/1
  io/1 -> abc to dq2/1
  abc to dq2/1 -> Demux2/1
  Demux2/3 -> Terminator2/1
  Gain1/1 -> Scope/1, w/1, Integrator/1
  Discrete Virtual PLL/2 -> Terminator4/1
  Demux2/1 -> pack6 Scope1/1, iod/1
  Demux2/2 -> pack6 Scope1/2, ioq/1

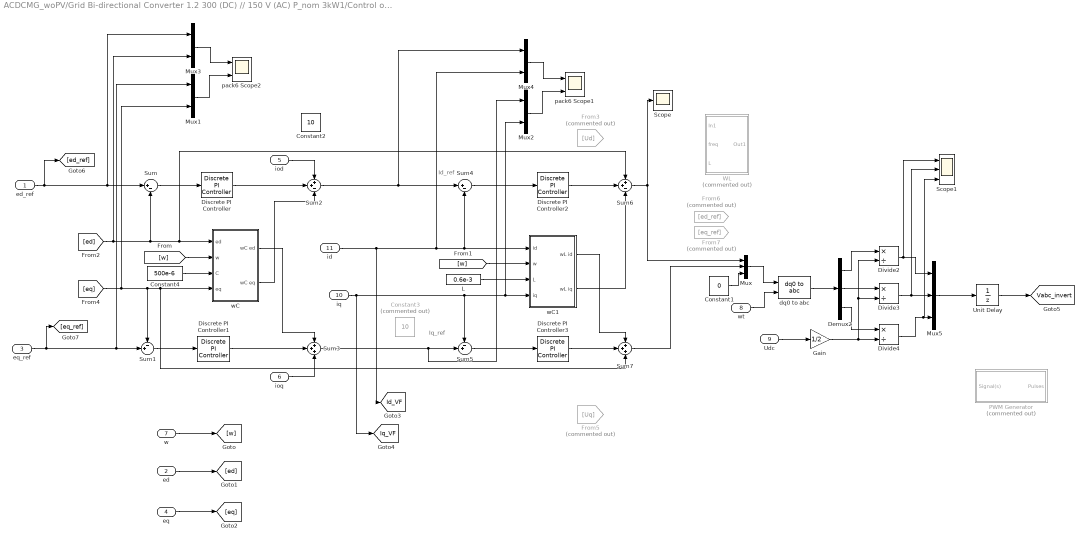
== system ACDCMG_woPV/Grid Bi-directional Converter 1.2 300 (DC) // 150 V (AC) P_nom 3kW1/Control of Inverter/V//F/UIcontrol ==
  note: Id_ref
  note: Iq_ref
  ed_ref : Inport
  ed : Inport  Port=2
  eq_ref : Inport  Port=3
  eq : Inport  Port=4
  iod : Inport  Port=5
  ioq : Inport  Port=6
  w : Inport  Port=7
  "wt " : Inport  Port=8
  Udc : Inport  Port=9
  iq : Inport  Port=10
  id : Inport  Port=11
  Constant1 : Constant  Value=0
  Constant2 : Constant  Value=10
  Constant3 : Constant  Commented=on  Value=10
  Constant4 : Constant  Value=500e-6
  Demux2 : Demux  Outputs=3
  Discrete PI Controller : powerlib_extras/Discrete  Control Blocks/Discrete PI Controller  Kp=5  Ki=50  Par_Limits=[1e6 -1e6]  Init=0  Ts=Ts_Control
  Discrete PI Controller1 : powerlib_extras/Discrete  Control Blocks/Discrete PI Controller  Kp=5  Ki=50  Par_Limits=[1e6 -1e6]  Init=0  Ts=Ts_Control
  Discrete PI Controller2 : powerlib_extras/Discrete  Control Blocks/Discrete PI Controller  Kp=25  Ki=1800  Par_Limits=[1e6 -1e6]  Init=0  Ts=Ts_Control
  Discrete PI Controller3 : powerlib_extras/Discrete  Control Blocks/Discrete PI Controller  Kp=25  Ki=1800  Par_Limits=[1e6 -1e6]  Init=0  Ts=Ts_Control
  Divide2 : Product  Inputs=*/
  Divide3 : Product  Inputs=*/
  Divide4 : Product  Inputs=*/
  From3 : From  Commented=on  GotoTag=Ud
  From5 : From  Commented=on  GotoTag=Uq
  From6 : From  Commented=on  GotoTag=ed_ref
  From7 : From  Commented=on  GotoTag=eq_ref
  Gain : Gain  Gain=1/2
  L : Constant  Value=0.6e-3
  Mux : Mux  Inputs=3
  Mux{1..4} (4 alike) : Mux  Inputs=2
  Mux5 : Mux  Inputs=3
  PWM Generator : Subsystem  Commented=on  AncestorBlock="powerlib_extras/Control  Blocks/PWM Generator"  DialogController=POWERSYS.PowerSysDialog  mask(PWM Generator){GeneratorMode=3-arm  bridge (6 pulses), Fc=10000, Internal=off, mIndex=0.4, Freq=50, Phase=0}
      mask prompts: GeneratorMode "Generator Mode"; Fc "Carrier frequency (Hz):"; Internal "Internal generation of modulating signal(s)"; mIndex "Modulation index  (0<m<1) :"; Freq "Frequency of output voltage (Hz)"; Phase "Phase of output voltage (degrees)"
      mask help:
      | This block generates pulses for carrier-based PWM (Pulse Width Modulation), self-commutated IGBTs,GTOs or FETs bridges.
      |
      | Depending on the number of bridge arms selected in the "Generator Mode" parameter, the block can be used either for single-phase or three-phase PWM control.
      mask init: same as ACDCMG_woPV/Grid Bi-directional Converter 1.2 300 (DC) // 150 V (AC) P_nom 3kW/Control of Inverter/V//F/UIcontrol/PWM Generator
      mask Help: web(psbhelp)
      mask TypeOptions GeneratorMode: 1-arm  bridge (2 pulses) | 2-arm  bridge (4 pulses) | 3-arm  bridge (6 pulses) | Double 3-arm  bridges (12 pulses)
      mask Callback Internal: p3=get_param(gcb,'Internal');if strcmp(p3,'on');visible={'on','on','on','on','on','on'};else;visible={'on','on','on','off','off','off'};end;set_param(gcb,'MaskVisibilities',visible)
  Scope : Scope
  Scope1 : Scope  NumInputPorts=3
  Sum : Sum  Inputs=|+-
  Sum1 : Sum  Inputs=-+|
  Sum2 : Sum  Inputs=++-
  Sum3 : Sum  Inputs=+++
  Sum4 : Sum  Inputs=|+-
  Sum5 : Sum  Inputs=-+|
  Sum6 : Sum  Inputs=++-
  Sum7 : Sum  Inputs=+++
  Unit Delay : UnitDelay  SampleTime=-1  HasFrameUpgradeWarning=on
  WL : Subsystem  Commented=on
  dq0 to abc : powerlib_meascontrol/Transformations/dq0 to abc  Alignment=90 degrees behind phase A axis
  pack6 Scope1 : Scope  NumInputPorts=2
  pack6 Scope2 : Scope  NumInputPorts=2
  wC : Subsystem
  wC1 : Subsystem
  tag scope: Id_VF=global, Iq_VF=global, Vabc_invert=global
  wires:
  ed_ref/1 -> [ed_ref], Mux3/1, Sum/1
  Sum/1 -> Discrete PI Controller/1
  Mux/1 -> dq0 to abc/1
  "wt "/1 -> dq0 to abc/2
  Mux5/1 -> Unit Delay/1
  Demux2/1 -> Divide2/1
  Demux2/2 -> Divide3/1
  Gain/1 -> Divide3/2, Divide2/2, Divide4/2
  Divide4/1 -> Scope1/3, Mux5/3
  Divide2/1 -> Mux5/1, Scope1/1
  Demux2/3 -> Divide4/1
  Divide3/1 -> Scope1/2, Mux5/2
  dq0 to abc/1 -> Demux2/1
  Udc/1 -> Gain/1
  Constant4/1 -> wC/3(C)
  [w] -> wC/2(w)
  [eq] -> Mux1/2, Sum7/3, wC/4(eq), Sum1/1
  Sum1/1 -> Discrete PI Controller1/1
  eq_ref/1 -> [eq_ref], Mux1/1, Sum1/2
  L/1 -> wC1/3(L)
  Sum5/1 -> Discrete PI Controller3/1
  Sum4/1 -> Discrete PI Controller2/1
  Discrete PI Controller3/1 -> Sum7/2
  Discrete PI Controller2/1 -> Sum6/2
  w/1 -> [w]
  [w] -> wC1/2(w)
  ed/1 -> [ed]
  eq/1 -> [eq]
  Sum6/1 -> Mux/1, Scope/1
  Constant1/1 -> Mux/3
  Mux4/1 -> pack6 Scope1/1
  Mux2/1 -> pack6 Scope1/2
  iq/1 -> [Iq_VF], Sum5/1, wC1/4(iq), Mux2/2
  Discrete PI Controller/1 -> Sum2/2
  Discrete PI Controller1/1 -> Sum3/2
  id/1 -> [Id_VF], Mux4/2, wC1/1(id), Sum4/2
  Mux3/1 -> pack6 Scope2/1
  Mux1/1 -> pack6 Scope2/2
  wC/1(wC ed) -> Sum3/1
  ioq/1 -> Sum3/3
  iod/1 -> Sum2/1
  wC/2(wC eq) -> Sum2/3
  wC1/1(wL id) -> Sum7/1
  wC1/2(wL iq) -> Sum6/3
  [ed] -> Sum6/1, wC/1(ed), Sum/2, Mux3/2
  Sum2/1 -> Mux4/1, Sum4/1
  Sum3/1 -> Mux2/1, Sum5/2
  Unit Delay/1 -> [Vabc_invert]
  Sum7/1 -> Mux/2

== system ACDCMG_woPV/Grid Bi-directional Converter 1.2 300 (DC) // 150 V (AC) P_nom 3kW1/Power Measurement (Three-Phase)/Continuous/Negative I2 ==
  Phasor_ABC : Inport
  Add : Sum  Inputs=+++
  Demux1 : Demux  Outputs=3
  Gain1 : Gain  Gain=1/3
  alpha : Gain  Gain=-0.5*(1-1j*sqrt(3))
  alpha2 : Gain  Gain=-0.5*(1+1j*sqrt(3))
  I2 : Outport  VectorParamsAs1DForOutWhenUnconnected=off
  wires:
  alpha/1 -> Add/3
  Demux1/3 -> alpha/1
  Demux1/2 -> alpha2/1
  alpha2/1 -> Add/2
  Add/1 -> Gain1/1
  Gain1/1 -> I2/1
  Demux1/1 -> Add/1
  Phasor_ABC/1 -> Demux1/1

== system ACDCMG_woPV/Grid Bi-directional Converter 1.2 300 (DC) // 150 V (AC) P_nom 3kW1/Power Measurement (Three-Phase)/Continuous/Negative V2 ==
  Phasor_ABC : Inport
  Add : Sum  Inputs=+++
  Demux1 : Demux  Outputs=3
  Gain1 : Gain  Gain=1/3
  alpha : Gain  Gain=-0.5*(1-1j*sqrt(3))
  alpha2 : Gain  Gain=-0.5*(1+1j*sqrt(3))
  V2 : Outport  VectorParamsAs1DForOutWhenUnconnected=off
  wires:
  Phasor_ABC/1 -> Demux1/1
  Demux1/1 -> Add/1
  Gain1/1 -> V2/1
  Add/1 -> Gain1/1
  alpha2/1 -> Add/2
  Demux1/2 -> alpha2/1
  Demux1/3 -> alpha/1
  alpha/1 -> Add/3

== system ACDCMG_woPV/Grid Bi-directional Converter 1.2 300 (DC) // 150 V (AC) P_nom 3kW1/Power Measurement (Three-Phase)/Continuous/Phase-A I ==
  Input : Inport
  SinCos : Inport  Port=2
  Demux : Demux  Outputs=2
  Gain : Gain  Gain=2*F
  Integrator : Integrator
  Product1 : Product
  Real-Imag to Complex : RealImagToComplex
  Subtract : Sum  Inputs=+-
  Transport Delay : TransportDelay  DelayTime=1/F  BufferSize=4096
  Phasor : Outport  VectorParamsAs1DForOutWhenUnconnected=off
  wires:
  Real-Imag to Complex/1 -> Phasor/1
  Subtract/1 -> Gain/1
  Product1/1 -> Integrator/1
  Integrator/1 -> Subtract/1, Transport Delay/1
  Demux/1 -> Real-Imag to Complex/1
  Gain/1 -> Demux/1
  Demux/2 -> Real-Imag to Complex/2
  Transport Delay/1 -> Subtract/2
  SinCos/1 -> Product1/2
  Input/1 -> Product1/1

== system ACDCMG_woPV/Grid Bi-directional Converter 1.2 300 (DC) // 150 V (AC) P_nom 3kW1/Power Measurement (Three-Phase)/Continuous/Phase-A V ==
  Input : Inport
  SinCos : Inport  Port=2
  Demux : Demux  Outputs=2
  Gain : Gain  Gain=2*F
  Integrator : Integrator
  Product1 : Product
  Real-Imag to Complex : RealImagToComplex
  Saturation : Saturate  UpperLimit=1  LowerLimit=-1
  Subtract : Sum  Inputs=+-
  Transport Delay : TransportDelay  DelayTime=1/F  BufferSize=4096
  Phasor : Outport  VectorParamsAs1DForOutWhenUnconnected=off
  wires:
  Input/1 -> Product1/1
  SinCos/1 -> Product1/2
  Transport Delay/1 -> Subtract/2
  Demux/2 -> Real-Imag to Complex/2
  Gain/1 -> Demux/1
  Demux/1 -> Real-Imag to Complex/1
  Integrator/1 -> Transport Delay/1, Subtract/1
  Subtract/1 -> Gain/1
  Real-Imag to Complex/1 -> Phasor/1
  Product1/1 -> Saturation/1
  Saturation/1 -> Integrator/1

== system ACDCMG_woPV/Grid Bi-directional Converter 1.2 300 (DC) // 150 V (AC) P_nom 3kW1/Power Measurement (Three-Phase)/Continuous/Phase-B I ==
  Input : Inport
  SinCos : Inport  Port=2
  Demux : Demux  Outputs=2
  Gain : Gain  Gain=2*F
  Integrator : Integrator
  Product1 : Product
  Real-Imag to Complex : RealImagToComplex
  Subtract : Sum  Inputs=+-
  Transport Delay : TransportDelay  DelayTime=1/F  BufferSize=4096
  Phasor : Outport  VectorParamsAs1DForOutWhenUnconnected=off
  wires:
  Input/1 -> Product1/1
  SinCos/1 -> Product1/2
  Transport Delay/1 -> Subtract/2
  Demux/2 -> Real-Imag to Complex/2
  Gain/1 -> Demux/1
  Demux/1 -> Real-Imag to Complex/1
  Integrator/1 -> Transport Delay/1, Subtract/1
  Product1/1 -> Integrator/1
  Subtract/1 -> Gain/1
  Real-Imag to Complex/1 -> Phasor/1
